simulink model "SimModel20260428"  (R2021b)
settings: Solver=VariableStepAuto  StartTime=0.0  StopTime=10.0  RelTol=1e-3
values from neighbouring files (symbols this model uses):
  Dall = 0.1    [parameter260428.m]
  Jall = 0.0177    [parameter260428.m]
  Kd = 100    [parameter260428.m]
  Ke = 0.0336    [parameter260428.m]
  Ki = 200    [parameter260428.m]
  Kp = 155    [parameter260428.m]
  Kt = 0.0223    [parameter260428.m]
  L = 0.000645    [parameter260428.m]
  MgLgamma = 0.00013    [parameter260428.m]
  R = 24.5    [parameter260428.m]
settings Model: Creator=higas  LastModifiedBy=higas

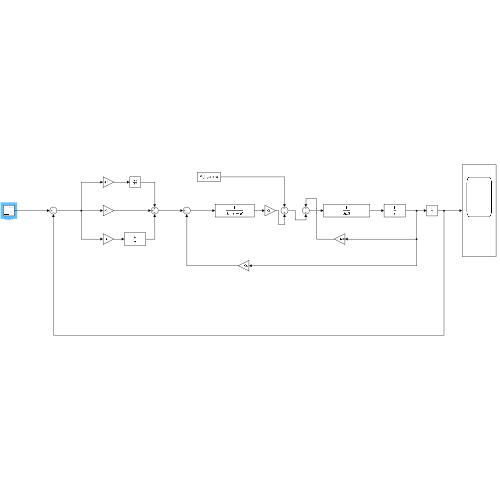
[thumbnail: Simulink's stored preview of the top-level diagram]
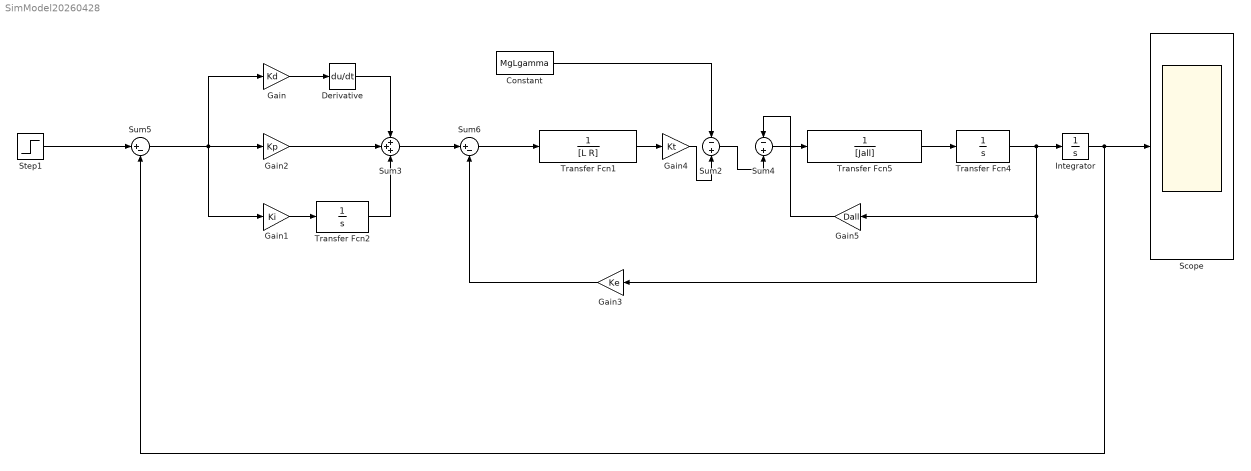
== system SimModel20260428 ==
  Constant : Constant  Value=MgLgamma
  Derivative : Derivative
  Gain : Gain  Gain=Kd
  Gain1 : Gain  Gain=Ki  RndMeth=Zero
  Gain2 : Gain  Gain=Kp
  Gain3 : Gain  Gain=Ke
  Gain4 : Gain  Gain=Kt
  Gain5 : Gain  Gain=Dall
  Integrator : Integrator
  Scope : Scope
  Step1 : Step  After=3.14  SampleTime=0
  Sum2 : Sum  Inputs=-+
  Sum3 : Sum  Inputs=+++
  Sum4 : Sum  Inputs=-+
  Sum5 : Sum  Inputs=|+-
  Sum6 : Sum  Inputs=|+-
  Transfer Fcn1 : TransferFcn  Denominator=[L R]
  Transfer Fcn2 : TransferFcn  Denominator=[1 0]
  Transfer Fcn4 : TransferFcn  Denominator=[1 0]
  Transfer Fcn5 : TransferFcn  Denominator=[Jall]
  wires:
  Gain/1 -> Derivative/1
  Derivative/1 -> Sum3/1
  Gain2/1 -> Sum3/2
  Gain1/1 -> Transfer Fcn2/1
  Transfer Fcn2/1 -> Sum3/3
  Integrator/1 -> Sum5/2, Scope/1
  Sum6/1 -> Transfer Fcn1/1
  Transfer Fcn1/1 -> Gain4/1
  Step1/1 -> Sum5/1
  Sum5/1 -> Gain1/1, Gain/1, Gain2/1
  Sum3/1 -> Sum6/1
  Transfer Fcn4/1 -> Gain3/1, Gain5/1, Integrator/1
  Constant/1 -> Sum2/1
  Gain4/1 -> Sum2/2
  Transfer Fcn5/1 -> Transfer Fcn4/1
  Sum4/1 -> Transfer Fcn5/1
  Sum2/1 -> Sum4/2
  Gain5/1 -> Sum4/1
  Gain3/1 -> Sum6/2
